simulink model "sim_control_two_input_two_output_linear_system"  (R2023a)
settings: Solver=VariableStepAuto  StartTime=0.0  StopTime=1  RelTol=1e-3
settings Model: Creator=ACCENT  LastModifiedBy=ACCENT

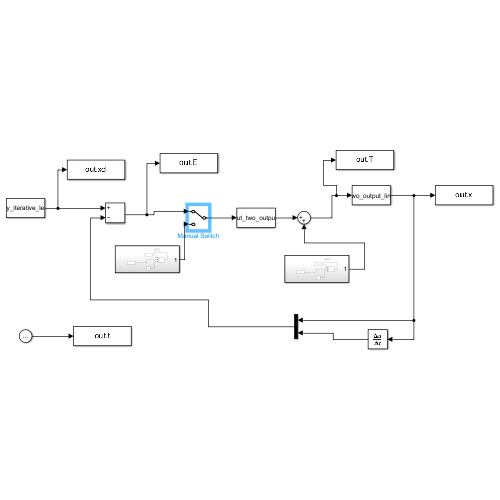
[thumbnail: Simulink's stored preview of the top-level diagram]
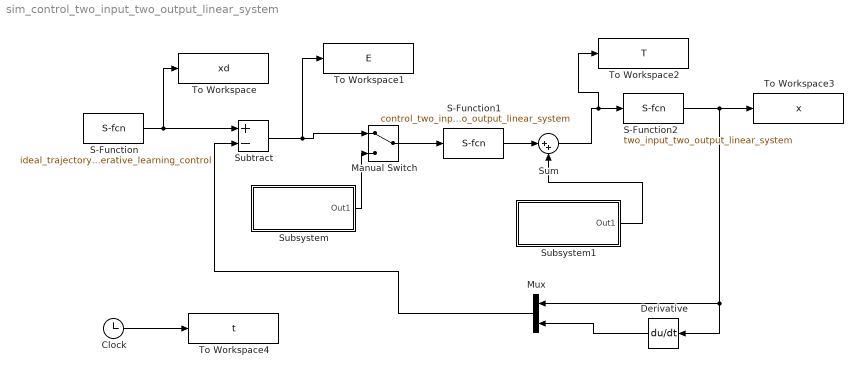
== system sim_control_two_input_two_output_linear_system ==
  Clock : Clock
  Derivative : Derivative
  Manual Switch : ManualSwitch
  Mux : Mux  Inputs=2
  S-Function : S-Function  FunctionName=ideal_trajectory_iterative_learning_control  SFunctionDeploymentMode=off  EnableBusSupport=off
  S-Function1 : S-Function  FunctionName=control_two_input_two_output_linear_system  SFunctionDeploymentMode=off  EnableBusSupport=off
  S-Function2 : S-Function  FunctionName=two_input_two_output_linear_system  SFunctionDeploymentMode=off  EnableBusSupport=off
  Subsystem : Subsystem
  Subsystem1 : Subsystem
  Subtract : Sum  Inputs=+-
  Sum : Sum  Inputs=|++
  To Workspace : ToWorkspace  VariableName=xd  SampleTime=0.01
  To Workspace1 : ToWorkspace  VariableName=E  SampleTime=0.01
  To Workspace2 : ToWorkspace  VariableName=T  SampleTime=0.01
  To Workspace3 : ToWorkspace  VariableName=x  SampleTime=0.01
  To Workspace4 : ToWorkspace  VariableName=t  SampleTime=0.01
  wires:
  Clock/1 -> To Workspace4/1
  S-Function/1 -> To Workspace/1, Subtract/1
  Subtract/1 -> To Workspace1/1, Manual Switch/1
  Subsystem/1(Out1) -> Manual Switch/2
  Manual Switch/1 -> S-Function1/1
  S-Function1/1 -> Sum/1
  Subsystem1/1(Out1) -> Sum/2
  Sum/1 -> To Workspace2/1, S-Function2/1
  S-Function2/1 -> Derivative/1, Mux/1, To Workspace3/1
  Derivative/1 -> Mux/2
  Mux/1 -> Subtract/2

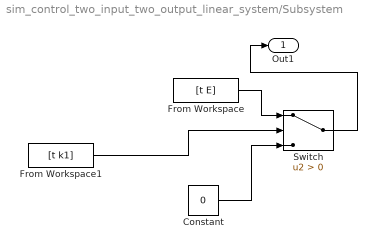
== system sim_control_two_input_two_output_linear_system/Subsystem ==
  Constant : Constant  Value=0
  From Workspace : FromWorkspace  VariableName=[t E]
  From Workspace1 : FromWorkspace  VariableName=[t k1]
  Switch : Switch  Criteria=u2 > Threshold  SaturateOnIntegerOverflow=off  InputSameDT=off
  Out1 : Outport
  wires:
  Switch/1 -> Out1/1
  From Workspace/1 -> Switch/1
  From Workspace1/1 -> Switch/2
  Constant/1 -> Switch/3

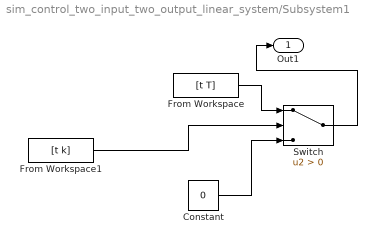
== system sim_control_two_input_two_output_linear_system/Subsystem1 ==
  Constant : Constant  Value=0
  From Workspace : FromWorkspace  VariableName=[t T]
  From Workspace1 : FromWorkspace  VariableName=[t k]
  Switch : Switch  Criteria=u2 > Threshold  SaturateOnIntegerOverflow=off  InputSameDT=off
  Out1 : Outport
  wires:
  Switch/1 -> Out1/1
  From Workspace1/1 -> Switch/2
  From Workspace/1 -> Switch/1
  Constant/1 -> Switch/3
